simulink model "ADCS_Outline"  (R2019a)
settings: Solver=VariableStepAuto  StartTime=0.0  StopTime=duration  MaxStep=step
InitFcn:
  | SC_ODIN_INITIALIZATION
values from neighbouring files (symbols this model uses):
  A = [ v(1) v(4) v(5) v(7);        v(4) v(2) v(6) v(8);        v(5) v(6) v(3) v(9);        v(7) v(8) v(9) v(10) ]    [MagnetometerCalibration.m]    (also in SC_ODIN_INITIALIZATION.m = 0.06; test.m = asin(sin(N)/sin(n)*sin(a)))
  Amag = [0.910186583854  -0.00959593267728  0.00343590491018; -0.00959593267728  1.05471221352  0.0559849466324; 0.00343590491018  0.0559849466324  1.05528532305]    [MagnetometerBias.mat]    (also in MagnetometerCalibration.m = evecs/scale*evecs')
  argentina = [1612.36;-4182.16;-4522.83]    [SC_ODIN_INITIALIZATION.m]
  As = 0.2*0.3    (= 0.06)    [SC_ODIN_INITIALIZATION.m]
  b_mag = block.InputPort(3).Data    [MagnetometerCalibration.m]    (also in SC_ODIN_INITIALIZATION.m = [10;-15.5;-12.2]*1e-6)
  bmag = [1.00003671399e-05 -1.55007781395e-05 -1.22009762149e-05]    [MagnetometerBias.mat]    (also in MagnetometerCalibration.m = centerE)
  breakpoints = data(:,1)    [SC_ODIN_INITIALIZATION.m]
  c = 2.99792458e8    (= 299792458)    [SC_ODIN_INITIALIZATION.m]
  C_I = [0.045 0.0009 -0.00007;        0.0009 0.045 -0.00003;        -0.00007 -0.00003 0.009]    [SC_ODIN_INITIALIZATION.m]
  Cd = 2.0    (= 2)    [SC_ODIN_INITIALIZATION.m]
  controller_sample_rate = 0.5    [SC_ODIN_INITIALIZATION.m]
  D = [ 2 * x,            2 * y,            2 * z,            1 + 0 * x ]    [MagnetometerCalibration.m]    (also in SC_ODIN_INITIALIZATION.m = 0.01*[1;1;1])
  datapx = data(:,2)    [SC_ODIN_INITIALIZATION.m]
  datapy = data(:,3)    [SC_ODIN_INITIALIZATION.m]
  datapz = data(:,4)    [SC_ODIN_INITIALIZATION.m]
  datavx = data(:,5)    [SC_ODIN_INITIALIZATION.m]
  datavy = data(:,6)    [SC_ODIN_INITIALIZATION.m]
  datavz = data(:,7)    [SC_ODIN_INITIALIZATION.m]
  DCM_BT0 = eye(3)    [SC_ODIN_INITIALIZATION.m]
  G = 6.67408e-11    [SC_ODIN_INITIALIZATION.m]
  ground = [1266.06;-4295.81;4526.14]    [SC_ODIN_INITIALIZATION.m]
  I = [Ixx -Ixy -Ixz;      -Ixy Iyy -Iyz;      -Ixz -Iyz Izz]    [SC_ODIN_INITIALIZATION.m]
  invA_mag = block.InputPort(2).Data    [MagnetometerCalibration.m]    (also in SC_ODIN_INITIALIZATION.m = inv(Ellrot/scale*Ellrot'))
  JD_0 = start_day+start_fraction    [SC_ODIN_INITIALIZATION.m]
  Ks = 1367    [SC_ODIN_INITIALIZATION.m]
  L = [0.0000812 -0.0022136 -0.0225868]    [SC_ODIN_INITIALIZATION.m]
  Ls = 0.01*[-3; 3; 5]    [SC_ODIN_INITIALIZATION.m]
  M = 5.9722e24    (= 5.9722e+24)    [SC_ODIN_INITIALIZATION.m]    (also in visualisation.m = uicontrol('Style','text','String',{''},'Position',[710 100+2)
  magnetorquer_tau = 0.02    [SC_ODIN_INITIALIZATION.m]
  magnetorquer_x_saturation = 0.24    [SC_ODIN_INITIALIZATION.m]
  magnetorquer_y_saturation = 0.24    [SC_ODIN_INITIALIZATION.m]
  magnetorquer_z_saturation = 0.13    [SC_ODIN_INITIALIZATION.m]
  namibia = [5659.26;1238.85;-2659.2]    [SC_ODIN_INITIALIZATION.m]
  q = 0.6    [SC_ODIN_INITIALIZATION.m]
  radii = radii .* sgns    [MagnetometerCalibration.m]    (also in SC_ODIN_INITIALIZATION.m = [1;0.9;1.1])
  W0 = [1;0;1-1/240].*pi()/180    [SC_ODIN_INITIALIZATION.m]
  wheel_saturation = 0.23e-3    (= 0.00023)    [SC_ODIN_INITIALIZATION.m]
  wheel_tau = 2    [SC_ODIN_INITIALIZATION.m]
undefined symbols (not defined in the file or in its folder): DiscIntNeverNeededParam, nut80, sun_sensors
libraries: dspmathops x94, vrlib x70, dspsrcs4 x21, realtime_pacer_lib x1, dspsolvers x1, dspinverses x1
(part 1 of 6)
settings Model: ExtModeTrigDuration=2  Creator=Charles  LastModifiedBy=erinp
settings SolverCC: MaxConsecutiveMinStep=2  ZeroCrossControl=DisableAll  ZeroCrossAlgorithm=Adaptive
settings DataIOCC: ReturnWorkspaceOutputs=off
settings OptimizationCC: DefaultParameterBehavior=Inlined  EnhancedBackFolding=on  PassReuseOutputArgsAs=Individual arguments  MaxStackSize=64  OptimizeBlockOrder=speed  DifferentSizesBufferReuse=on  OptimizationCustomize=off
settings DebuggingCC: ReadBeforeWriteMsg=DisableAll  WriteAfterWriteMsg=DisableAll  WriteAfterReadMsg=DisableAll  IgnoredZcDiagnostic=none  MultiTaskDSMMsg=none  ParameterTunabilityLossMsg=error  ArithmeticOperatorsInVariantConditions=warning
settings HardwareCC: ProdBitPerInt=16  ProdBitPerPointer=16  ProdBitPerSizeT=16  ProdBitPerPtrDiffT=16  ProdLargestAtomicFloat=None  ProdWordSize=8  ProdHWDeviceType=Atmel->AVR  UseEmbeddedCoderFeatures=off  UseSimulinkCoderFeatures=off
settings ModelReferenceCC: UpdateModelReferenceTargets=IfOutOfDate
settings SFSimCC: SFSimEcho=off  MATLABDynamicMemAlloc=off
settings RTWCC: SystemTargetFile=ert.tlc  TemplateMakefile=ert_default_tmf  GenerateReport=on  Toolchain=Arduino AVR  BuildConfiguration=Faster Runs  IncludeHyperlinkInReport=on  LaunchReport=on  GenerateTraceInfo=on  GenerateTraceReport=on  GenerateTraceReportSl=on  GenerateTraceReportSf=on  GenerateTraceReportEml=on
settings CodeAppCC: ForceParamTrailComments=on  IgnoreCustomStorageClasses=off  OperatorAnnotations=on  SimulinkDataObjDesc=on  SFDataObjDesc=on  InsertBlockDesc=on
settings ERTTargetCC: SupportContinuousTime=on  SupportNonInlinedSFcns=on  ERTCustomFileTemplate=example_file_process.tlc

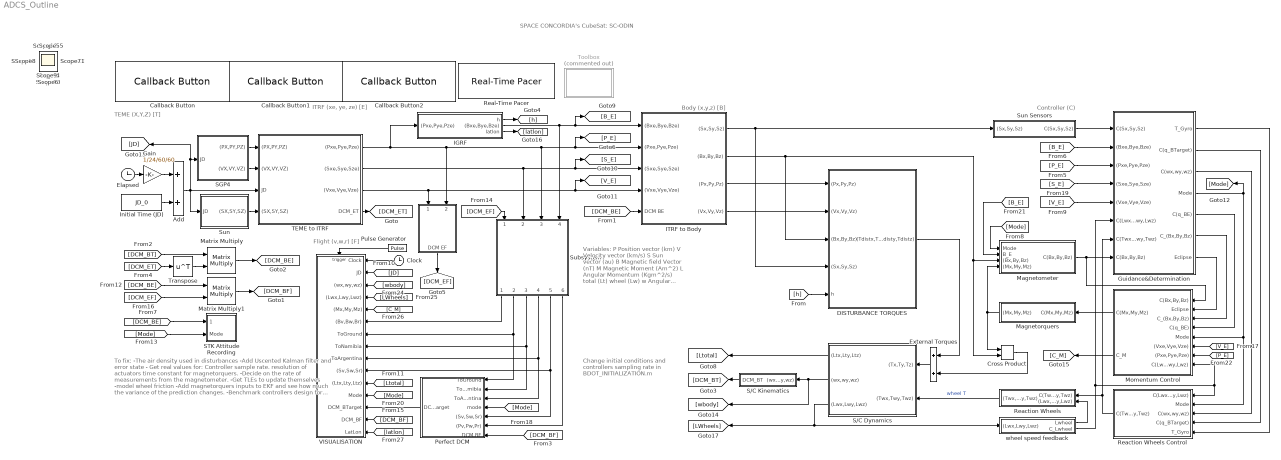
== system ADCS_Outline ==
  note: To fix:
      | -The air density used in disturbances
      | -Add Uscented Kalman filter and error state
      | - Get real values for:
      | Controller sample rate.
      | resolution of actuators
      | time constant for magnetorquers.
      | -Decide on the rate of measurements from the magnetometer.
      | -Get TLEs to update themselves
      | -model wheel friction
      | -Add magnetorquers inputs to EKF and see how much the variance of the prediction changes.
      | -Benchmark controllers design for other mission and see if ours makes sense.
      | -Get better estimate for center of mass from the Mech team
      | -Model vibrations from RWs with Vibs team
      | Stability: 0.01s picture. pixel = 3.2e-6 degrees
      |
      | -
      | -
  note: SPACE CONCORDIA's CubeSat: SC-ODIN
  note: Controller (C)
  note: Change initial conditions and controllers sampling rate in BDOT_INITIALIZATION.m
  note: Body (x,y,z) [B]
  note: Variables:
      |
      | P Position vector (km)
      | V Velocity vector (km/s)
      | S Sun vector (au)
      | B Magnetic field Vector (nT)
      | M Magnetic Moment (Am^2)
      | L Angular Momentum (Kgm^2/s)
      | total (Lt)
      | wheel (Lw)
      | w Angular velocity (rad/s)
      | T torque (Nm)
      | h Height from ground (km)
      | DCM Direction Cosine Matrix
  note: Flight (v,w,r) [F]
  note: TEME (X,Y,Z) [T]
  note: ITRF (xe, ye, ze) [E]
  "   " : Subsystem
  Add : Sum
  Callback Button : CallbackButton  ButtonText=Exclude visual
      settings: ClickFcn=|
      | if strcmp(get_param('ADCS_Outline/Callback Button','ButtonText'),'Include visual')
      | %un-comment visual related blocks
      | set_param('ADCS_Outline/Perfect DCM','Commented','off')
      | set_param('ADCS_Outline/VISUALISATION','Commented','off')
      | set_param('ADCS_Outline/From10','Commented','off')
      | set_param('ADCS_Outline/From11','Commented','off')
      | set_param('ADCS_Outline/From20','Commented','off')
      | set_param('ADCS_Outline/From15','Commented','off')
      | set_param('ADCS_Outline/From18','Commented','off')
      | set_param('ADCS_Outline/From3','Commented','off')
      | set_param('ADCS_Outline/   ','Commented','off')
      | set_param('ADCS_Outline/Goto5','Commented','off')
      | set_param('ADCS_Outline/Subsystem1','Commented','off')
      | set_param('ADCS_Outline/Subsystem1','Commented','off')
      | set_param('ADCS_Outline/Goto8','Commented','off')
      | set_param('ADCS_Outline/Matrix Multiply1','Commented','off')
      | set_param('ADCS_Outline/From12','Commented','off')
      | set_param('ADCS_Outline/From16','Commented','off')
      | set_param('ADCS_Outline/Goto1','Commented','off')
      | set_param('ADCS_Outline/From14','Commented','off')
      | set_param('ADCS_Outline/Goto13','Commented','off')
      | set_param('ADCS_Outline/From24','Commented','off')
      | set_param('ADCS_Outline/From25','Commented','off')
      | set_param('ADCS_Outline/From26','Commented','off')
      | set_param('ADCS_Outline/From27','Commented','off')
      | set_param('ADCS_Outline/Clock','Commented','off')
      | set_param('ADCS_Outline/Pulse Generator','Commented','off')
      | set_param('ADCS_Outline/Goto14','Commented','off')
      | set_param('ADCS_Outline/Goto15','Commented','off')
      | set_param('ADCS_Outline/Goto16','Commented','off')
      | set_param('ADCS_Outline/Goto17','Commented','off')
      | 
      | %change button text
      | set_param('ADCS_Outline/Callback Button','ButtonText','Exclude visual')
      | 
      | else
      | %comments out visual related blocks
      | set_param('ADCS_Outline/Perfect DCM','Commented','on')
      | set_param('ADCS_Outline/VISUALISATION','Commented','on')
      | set_param('ADCS_Outline/From10','Commented','on')
      | set_param('ADCS_Outline/From11','Commented','on')
      | set_param('ADCS_Outline/From20','Commented','on')
      | set_param('ADCS_Outline/From15','Commented','on')
      | set_param('ADCS_Outline/From18','Commented','on')
      | set_param('ADCS_Outline/From3','Commented','on')
      | set_param('ADCS_Outline/   ','Commented','on')
      | set_param('ADCS_Outline/Goto5','Commented','on')
      | set_param('ADCS_Outline/Subsystem1','Commented','on')
      | set_param('ADCS_Outline/Subsystem1','Commented','on')
      | set_param('ADCS_Outline/Goto8','Commented','on')
      | set_param('ADCS_Outline/Matrix Multiply1','Commented','on')
      | set_param('ADCS_Outline/From12','Commented','on')
      | set_param('ADCS_Outline/From16','Commented','on')
      | set_param('ADCS_Outline/Goto1','Commented','on')
      | set_param('ADCS_Outline/From14','Commented','on')
      | set_param('ADCS_Outline/Goto13','Commented','on')
      | set_param('ADCS_Outline/From24','Commented','on')
      | set_param('ADCS_Outline/From25','Commented','on')
      | set_param('ADCS_Outline/From26','Commented','on')
      | set_param('ADCS_Outline/From27','Commented','on')
      | set_param('ADCS_Outline/Clock','Commented','on')
      | set_param('ADCS_Outline/Pulse Generator','Commented','on')
      | set_param('ADCS_Outline/Goto14','Commented','on')
      | set_param('ADCS_Outline/Goto15','Commented','on')
      | set_param('ADCS_Outline/Goto16','Commented','on')
      | set_param('ADCS_Outline/Goto17','Commented','on')
      | 
      | %change button text
      | set_param('ADCS_Outline/Callback Button','ButtonText','Include visual')
      | end
  Callback Button1 : CallbackButton  ButtonText=Exclude STK Recording
      settings: ClickFcn=|
      | if strcmp(get_param('ADCS_Outline/Callback Button1','ButtonText'),'Include STK Recording')
      | %un-comment visual related blocks
      | set_param('ADCS_Outline/From7','Commented','off')
      | set_param('ADCS_Outline/From13','Commented','off')
      | set_param('ADCS_Outline/STK Attitude Recording','Commented','off')
      | 
      | %change button text
      | set_param('ADCS_Outline/Callback Button1','ButtonText','Exclude STK Recording')
      | 
      | else
      | %comments out visual related blocks
      | set_param('ADCS_Outline/From7','Commented','on')
      | set_param('ADCS_Outline/From13','Commented','on')
      | set_param('ADCS_Outline/STK Attitude Recording','Commented','on')
      | 
      | %change button text
      | set_param('ADCS_Outline/Callback Button1','ButtonText','Include STK Recording')
      | end
  Callback Button2 : CallbackButton  ButtonText=Exclude Momentum
      settings: ClickFcn=|
      | if strcmp(get_param('ADCS_Outline/Callback Button2','ButtonText'),'Include Momentum')
      | %un-comment visual related blocks
      | set_param('ADCS_Outline/Momentum Control','Commented','off')
      | set_param('ADCS_Outline/Magnetorquers','Commented','off')
      | set_param('ADCS_Outline/DISTURBANCE TORQUES','Commented','off')
      | set_param('ADCS_Outline/Cross Product','Commented','off')
      | set_param('ADCS_Outline/External Torques','Commented','off')
      | set_param('ADCS_Outline/From','Commented','off')
      | set_param('ADCS_Outline/Goto4','Commented','off')
      | 
      | %change button text
      | set_param('ADCS_Outline/Callback Button2','ButtonText','Exclude Momentum')
      | 
      | else
      | %comments out visual related blocks
      | set_param('ADCS_Outline/Momentum Control','Commented','on')
      | set_param('ADCS_Outline/Magnetorquers','Commented','on')
      | set_param('ADCS_Outline/DISTURBANCE TORQUES','Commented','on')
      | set_param('ADCS_Outline/Cross Product','Commented','on')
      | set_param('ADCS_Outline/External Torques','Commented','on')
      | set_param('ADCS_Outline/From','Commented','on')
      | set_param('ADCS_Outline/Goto4','Commented','on')
      | 
      | %change button text
      | set_param('ADCS_Outline/Callback Button2','ButtonText','Include Momentum')
      | end
  Clock : Clock
  Cross Product : vrlib/Utilities/Cross Product
      settings: SourceProductBaseCode=VR
  DISTURBANCE TORQUES : Subsystem
  Elapsed : Clock
  External Torques : Sum
  Gain : Gain  Gain=1/24/60/60
  Guidance&Determination : Subsystem  TreatAsAtomicUnit=on  SystemSampleTime=controller_sample_rate
  IGRF : Subsystem
  ITRF to Body : Subsystem
  Initial Time (JD) : Constant  Value=JD_0
  "Magnetometer " : Subsystem  TreatAsAtomicUnit=on  SystemSampleTime=controller_sample_rate
  Magnetorquers : Subsystem
  Matrix Multiply : Product  Multiplication=Matrix(*)
  Matrix Multiply1 : Product  Multiplication=Matrix(*)
  Momentum Control : Subsystem  TreatAsAtomicUnit=on  SystemSampleTime=controller_sample_rate/2
  Perfect DCM : Subsystem
  Pulse Generator : DiscretePulseGenerator  PulseType=Time based  Period=1  PulseWidth=5
  Reaction Wheels : Subsystem
  Reaction Wheels Control : Subsystem  TreatAsAtomicUnit=on  SystemSampleTime=controller_sample_rate
  Real-Time Pacer : realtime_pacer_lib/Real-Time Pacer  simTimePerRealTime=inf
  S/C Dynamics : Subsystem
  S/C Kinematics : Subsystem
  SGP4 : Subsystem
  STK Attitude Recording : Subsystem  StopFcn=STKAttitudeFileGenerator
  Subsystem1 : Subsystem
  Sun : Subsystem
  Sun Sensors : Subsystem  TreatAsAtomicUnit=on  SystemSampleTime=controller_sample_rate
  TEME to ITRF : Subsystem
  Toolbox : Subsystem  Commented=on
  Transpose : Math  Operator=transpose  SaturateOnIntegerOverflow=on
  VISUALISATION : Subsystem
  wheel speed feedback : Subsystem
  Scope{,1..10,12..21} (21 alike) : Scope
  wires:
  DISTURBANCE TORQUES/1((Tdistx,Tdisty,Tdistz)) -> External Torques/1
  ITRF to Body/3((Px,Py,Pz)) -> DISTURBANCE TORQUES/1((Px,Py,Pz))
  TEME to ITRF/3((Vxe,Vye,Vze)) -> ITRF to Body/4((Vxe,Vye,Vze)), [V_E], "   "/1((Vxe,Xye,Vze))
  Elapsed/1 -> Gain/1
  Gain/1 -> Add/1
  External Torques/1 -> S/C Dynamics/1((Tx,Ty,Tz))
  Initial Time (JD)/1 -> Add/2
  SGP4/2((VX,VY,VZ)) -> TEME to ITRF/2((VX,VY,VZ))
  SGP4/1((PX,PY,PZ)) -> TEME to ITRF/1((PX,PY,PZ))
  TEME to ITRF/2((Sxe,Sye,Sze)) -> ITRF to Body/3((Sxe,Sye,Sze)), [S_E], Subsystem1/2((Sxe,Sye,Sze))
  TEME to ITRF/4(DCM_ET) -> [DCM_ET]
  Matrix Multiply/1 -> [DCM_BE]
  IGRF/1("h ") -> [h]
  [h] -> DISTURBANCE TORQUES/5(h)
  [DCM_BT] -> Matrix Multiply/1
  [DCM_ET] -> Transpose/1
  Transpose/1 -> Matrix Multiply/2
  ITRF to Body/4((Vx,Vy,Vz)) -> DISTURBANCE TORQUES/2((Vx,Vy,Vz))
  TEME to ITRF/1((Pxe,Pye,Pze)) -> Subsystem1/3((Pxe,Pye,Pze)), ITRF to Body/2((Pxe,Pye,Pze)), [P_E], "   "/2((Pxe,Pye,Pze)), IGRF/1((Pxe,Pye,Pze))
  IGRF/2((Bxe,Bye,Bze)) -> Subsystem1/4((Bxe,Bye,Bze)), ITRF to Body/1((Bxe,Bye,Bze)), [B_E]
  Cross Product/1 -> External Torques/2
  Reaction Wheels Control/1(C(Twx,Twy,Twz)) -> Reaction Wheels/1(C(Twx,Twy,Twz)), Guidance&Determination/7(C(Twx,Twy,Twz))
  Reaction Wheels/1((Twx,Twy,Twz)) -> S/C Dynamics/2((Twx,Twy,Twz))  "wheel T"
  S/C Dynamics/3((Lwx,Lwy,Lwz)) -> wheel speed feedback/1((Lwx,Lwy,Lwz)), [LWheels]
  S/C Dynamics/1((Ltx,Lty,Ltz)) -> [Ltotal]
  "   "/1(DCM EF) -> [DCM_EF]
  [Ltotal] -> VISUALISATION/11((Ltx,Lty,Ltz))
  Momentum Control/1(C(Mx,My,Mz)) -> Magnetorquers/1(C(Mx,My,Mz))
  [DCM_EF] -> Matrix Multiply1/2
  [DCM_BE] -> Matrix Multiply1/1
  Matrix Multiply1/1 -> [DCM_BF]
  [DCM_EF] -> Subsystem1/1("DCM_EF ")
  [JD] -> VISUALISATION/2(JD)
  Subsystem1/1((Bv,Bw,Br)) -> VISUALISATION/6((Bv,Bw,Br))
  Sun Sensors/1(C(Sx,Sy,Sz)) -> Guidance&Determination/1(C(Sx,Sy,Sz))
  Subsystem1/2(ToGround) -> Perfect DCM/1(ToGround), VISUALISATION/7(ToGround)
  Subsystem1/5((Sv,Sw,Sr)) -> Perfect DCM/5((Sv,Sw,Sr)), VISUALISATION/10((Sv,Sw,Sr))
  [DCM_BF] -> VISUALISATION/14(DCM_BF)
  Sun/1((SX,SY,SZ)) -> TEME to ITRF/4((SX,SY,SZ))
  Perfect DCM/1(DCM BTarget) -> VISUALISATION/13(DCM_BTarget)
  [DCM_BF] -> Perfect DCM/7(DCM BF)
  Guidance&Determination/4(Mode) -> Reaction Wheels Control/2(Mode), Momentum Control/5(Mode), [Mode]
  [Mode] -> VISUALISATION/12(Mode)
  wheel speed feedback/2(C_Lwheel) -> Guidance&Determination/6(C(Lwx,Lwy,Lwz)), Momentum Control/8(C(Lwx,Lwy,Lwz)), Reaction Wheels Control/1(C(Lwx,Lwy,Lwz))
  Subsystem1/4(ToArgentina) -> Perfect DCM/3(ToArgentina), VISUALISATION/9(ToArgentina)
  Add/1 -> Sun/1(JD), SGP4/1(JD), [JD], TEME to ITRF/3(JD)
  [DCM_BE] -> STK Attitude Recording/1(DCM_BE)
  Subsystem1/3(ToNamibia) -> Perfect DCM/2(ToNamibia), VISUALISATION/8(ToNamibia)
  Subsystem1/6((Pv,Pw,Pr)) -> Perfect DCM/6((Pv,Pw,Pr))
  ITRF to Body/2((Bx,By,Bz)) -> DISTURBANCE TORQUES/3((Bx,By,Bz)), Cross Product/2, "Magnetometer "/3((Bx,By,Bz))
  Guidance&Determination/3(C(wx,wy,wz)) -> Reaction Wheels Control/3(C(wx,wy,wz))
  [Mode] -> STK Attitude Recording/2(Mode)
  ITRF to Body/1((Sx,Sy,Sz)) -> Sun Sensors/1((Sx,Sy,Sz)), DISTURBANCE TORQUES/4((Sx,Sy,Sz))
  [Mode] -> Perfect DCM/4(mode)
  [V_E] -> Momentum Control/6((Vxe,Vye,Vze))
  [P_E] -> Momentum Control/7((Pxe,Pye,Pze))
  [wbody] -> VISUALISATION/3((wx,wy,wz))
  [LWheels] -> VISUALISATION/4((Lwx,Lwy,Lwz))
  [C_M] -> VISUALISATION/5((Mx,My,Mz))
  Magnetorquers/1((Mx,My,Mz)) -> "Magnetometer "/4((Mx,My,Mz)), Cross Product/1
  Momentum Control/2(C_M) -> [C_M]
  IGRF/3(latlon) -> [latlon]
  [latlon] -> VISUALISATION/15(LatLon)
  Pulse Generator/1 -> VISUALISATION/Trigger
  Clock/1 -> VISUALISATION/1(Clock)
  Guidance&Determination/2(C(q_BTarget)) -> Reaction Wheels Control/4(C(q_BTarget))
  Guidance&Determination/5(C(q_BE)) -> Momentum Control/4(C(q_BE))
  Guidance&Determination/6(C_(Bx,By,Bz)) -> Momentum Control/3(C_(Bx,By,Bz))
  "Magnetometer "/1(C(Bx,By,Bz)) -> Guidance&Determination/8(C(Bx,By,Bz)), Momentum Control/1(C(Bx,By,Bz))
  wheel speed feedback/1(Lwheel) -> Reaction Wheels/2((Lwx,Lwy,Lwz))
  [Mode] -> "Magnetometer "/1(Mode)
  S/C Kinematics/1(DCM_BT) -> [DCM_BT]
  Guidance&Determination/7(Eclipse) -> Momentum Control/2(Eclipse)
  S/C Dynamics/2((wx,wy,wz)) -> S/C Kinematics/1(" (wx,wy,wz)"), [wbody]
  [DCM_BE] -> ITRF to Body/5(DCM BE)
  [B_E] -> "Magnetometer "/2(B_E)
  [B_E] -> Guidance&Determination/2((Bxe,Bye,Bze))
  [P_E] -> Guidance&Determination/3((Pxe,Pye,Pze))
  [S_E] -> Guidance&Determination/4((Sxe,Sye,Sze))
  [V_E] -> Guidance&Determination/5((Vxe,Vye,Vze))
  Guidance&Determination/1(T_Gyro) -> Reaction Wheels Control/5(T_Gyro)

== system ADCS_Outline/    ==
  (Vxe,Xye,Vze) : Inport
  (Pxe,Pye,Pze) : Inport  Port=2
  Constant : Constant  Value=[1;0;0]
  Constant1 : Constant  Value=[0;0;1]
  Cross Product{,1..3} (4 alike) : vrlib/Utilities/Cross Product
      settings: SourceProductBaseCode=VR
  Matrix Concatenate : Concatenate  NumInputs=3  Mode=Multidimensional array  ConcatenateDimension=2
  Matrix Concatenate1 : Concatenate  NumInputs=3  Mode=Multidimensional array  ConcatenateDimension=2
  Matrix Multiply : Product  Multiplication=Matrix(*)
  Normalization{,1..5} (6 alike) : dspmathops/Normalization  NormType=2-norm  Bias=1e-10  NormOver=Each column  Dimension=1  roundingMode=Floor  overflowMode=off  accumDataTypeStr=Inherit: Same as product output  accumLastDataTypeStr=Inherit: Same as product output  outputDataTypeStr=Inherit: Same as product output  outputMin=[]  outputMax=[]  outputLastDataTypeStr=Inherit: Same as product output
      settings: SourceProductName=DSP System Toolbox
  Signal Specification1 : SignalSpecification  Dimensions=3
  Transpose : Math  Operator=transpose  SaturateOnIntegerOverflow=on
  DCM EF : Outport
  wires:
  Normalization/1 -> Matrix Concatenate/3, Cross Product1/1
  Normalization5/1 -> Matrix Concatenate1/1, Cross Product3/2
  Cross Product1/1 -> Normalization1/1
  Normalization3/1 -> Matrix Concatenate1/2
  Cross Product3/1 -> Signal Specification1/1
  Constant1/1 -> Cross Product/2
  Normalization4/1 -> Matrix Concatenate/1, Cross Product1/2
  Constant/1 -> Normalization4/1, Cross Product/1
  Cross Product2/1 -> Normalization2/1
  Cross Product/1 -> Normalization/1
  Normalization1/1 -> Matrix Concatenate/2
  Normalization2/1 -> Cross Product3/1, Matrix Concatenate1/3
  Matrix Concatenate/1 -> Transpose/1
  Matrix Concatenate1/1 -> Matrix Multiply/1
  Transpose/1 -> Matrix Multiply/2
  (Vxe,Xye,Vze)/1 -> Cross Product2/1, Normalization5/1
  (Pxe,Pye,Pze)/1 -> Cross Product2/2
  Matrix Multiply/1 -> DCM EF/1
  Signal Specification1/1 -> Normalization3/1

== system ADCS_Outline/DISTURBANCE TORQUES ==
  note: DISTURBANCE TORQUE
  (Px,Py,Pz) : Inport
  (Vx,Vy,Vz) : Inport  Port=2
  (Bx,By,Bz) : Inport  Port=3
  (Sx,Sy,Sz) : Inport  Port=4
  h : Inport  Port=5
  ATMOSPHERIC DRAG : Subsystem
  GRAVITY GRADIENT : Subsystem
  Inertia Matrix : Constant  Value=I
  "MAGNETIC FIELD " : Subsystem
  S/C residual Dipole Moment : Constant  Value=D
  SOLAR RADIATION PRESSURE : Subsystem
  Scope : Scope  NumInputPorts=4
  Sum : Sum  Inputs=++++
  (Tdistx,Tdisty,Tdistz) : Outport
  wires:
  (Px,Py,Pz)/1 -> GRAVITY GRADIENT/1((px,py,pz))
  (Sx,Sy,Sz)/1 -> SOLAR RADIATION PRESSURE/1((Sx,Sy,Sz))
  Inertia Matrix/1 -> GRAVITY GRADIENT/2("(Ixx Ixy Ixz, Iyx Iyy Iyz, Izx Izy Izz)")
  (Vx,Vy,Vz)/1 -> ATMOSPHERIC DRAG/1((vx,vy,vz))
  (Bx,By,Bz)/1 -> "MAGNETIC FIELD "/2((Bx,By,Bz))
  S/C residual Dipole Moment/1 -> "MAGNETIC FIELD "/1((Dx,Dy,Dz))
  "MAGNETIC FIELD "/1((Tmx,Tmy,Tmz)) -> Scope/1, Sum/1
  GRAVITY GRADIENT/1((Tgx,Tgy,Tgz)) -> Scope/2, Sum/2
  SOLAR RADIATION PRESSURE/1("(Tsx,Tsy, Tsz)") -> Scope/3, Sum/3
  ATMOSPHERIC DRAG/1((Tax,Tay,Taz)) -> Scope/4, Sum/4
  h/1 -> ATMOSPHERIC DRAG/2("h ")
  Sum/1 -> (Tdistx,Tdisty,Tdistz)/1

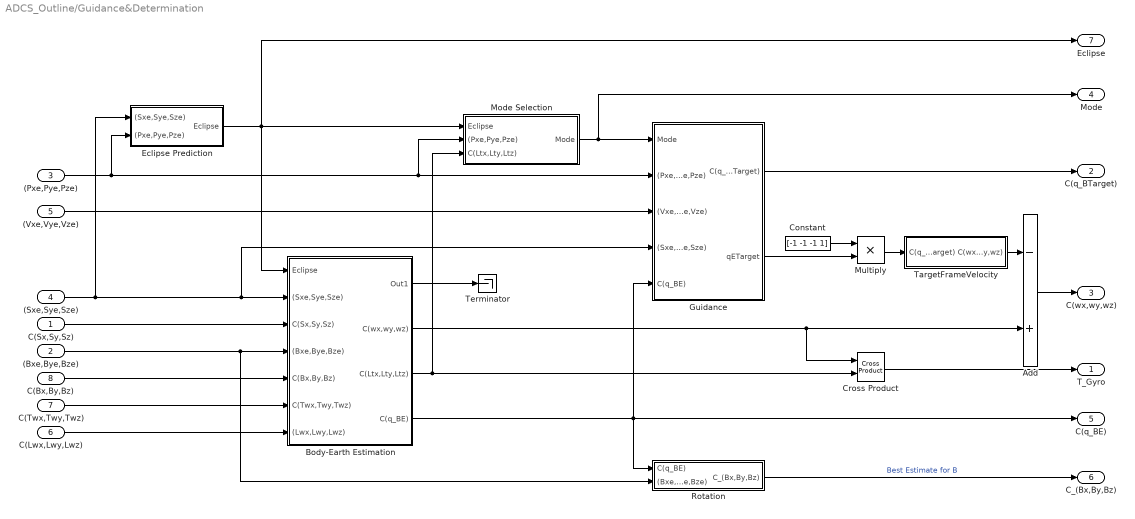
== system ADCS_Outline/Guidance&Determination ==
  C(Sx,Sy,Sz) : Inport
  (Bxe,Bye,Bze) : Inport  Port=2
  (Pxe,Pye,Pze) : Inport  Port=3
  (Sxe,Sye,Sze) : Inport  Port=4
  (Vxe,Vye,Vze) : Inport  Port=5
  C(Lwx,Lwy,Lwz) : Inport  Port=6
  C(Twx,Twy,Twz) : Inport  Port=7
  C(Bx,By,Bz) : Inport  Port=8
  Add : Sum  Inputs=-+
  Body-Earth Estimation : Subsystem
  Constant : Constant  Value=[-1 -1 -1 1]
  Cross Product : vrlib/Utilities/Cross Product
      settings: SourceProductBaseCode=VR
  Eclipse Prediction : Subsystem
  Guidance : Subsystem
  Mode Selection : Subsystem
  Multiply : Product
  Rotation : Subsystem
  TargetFrameVelocity : Subsystem
  Terminator : Terminator
  T_Gyro : Outport
  C(q_BTarget) : Outport  Port=2
  C(wx,wy,wz) : Outport  Port=3
  Mode : Outport  Port=4
  C(q_BE) : Outport  Port=5
  C_(Bx,By,Bz) : Outport  Port=6
  Eclipse : Outport  Port=7
  wires:
  (Bxe,Bye,Bze)/1 -> Body-Earth Estimation/4((Bxe,Bye,Bze)), Rotation/2((Bxe,Bye,Bze))
  (Sxe,Sye,Sze)/1 -> Eclipse Prediction/1((Sxe,Sye,Sze)), Guidance/4((Sxe,Sye,Sze)), Body-Earth Estimation/2((Sxe,Sye,Sze))
  (Pxe,Pye,Pze)/1 -> Eclipse Prediction/2((Pxe,Pye,Pze)), Mode Selection/2((Pxe,Pye,Pze)), Guidance/2((Pxe,Pye,Pze))
  C(Lwx,Lwy,Lwz)/1 -> Body-Earth Estimation/7((Lwx,Lwy,Lwz))
  C(Sx,Sy,Sz)/1 -> Body-Earth Estimation/3(C(Sx,Sy,Sz))
  C(Twx,Twy,Twz)/1 -> Body-Earth Estimation/6(C(Twx,Twy,Twz))
  Body-Earth Estimation/4(C(q_BE)) -> Guidance/5(C(q_BE)), C(q_BE)/1, Rotation/1(C(q_BE))
  (Vxe,Vye,Vze)/1 -> Guidance/3((Vxe,Vye,Vze))
  Guidance/1(C(q_BTarget)) -> C(q_BTarget)/1
  Mode Selection/1(Mode) -> Mode/1, Guidance/1(Mode)
  Body-Earth Estimation/3(C(Ltx,Lty,Ltz)) -> Mode Selection/3(C(Ltx,Lty,Ltz)), Cross Product/2
  Rotation/1(C_(Bx,By,Bz)) -> C_(Bx,By,Bz)/1  "Best Estimate for B"
  C(Bx,By,Bz)/1 -> Body-Earth Estimation/5(C(Bx,By,Bz))
  Eclipse Prediction/1(Eclipse) -> Body-Earth Estimation/1(Eclipse), Eclipse/1, Mode Selection/1(Eclipse)
  Add/1 -> C(wx,wy,wz)/1
  Body-Earth Estimation/2(C(wx,wy,wz)) -> Cross Product/1, Add/2
  Constant/1 -> Multiply/1
  Guidance/2(qETarget) -> Multiply/2
  TargetFrameVelocity/1(C(wx,wy,wz)) -> Add/1
  Multiply/1 -> TargetFrameVelocity/1(C(q_ETarget))
  Body-Earth Estimation/1(Out1) -> Terminator/1
  Cross Product/1 -> T_Gyro/1

== system ADCS_Outline/IGRF ==
  note: NED (n,e,d)
  (Pxe,Pye,Pze) : Inport
  Demux : Demux  Outputs=3
  Dot Product : DotProduct  InputSameDT=on  OutDataTypeStr=Inherit: Inherit via internal rule
  Gain : Gain  Gain=-1
  Gain1 : Gain  Gain=1e-9
  MATLAB Function : MATLAB Function  TreatAsAtomicUnit=on
  MATLAB Function1 : MATLAB Function  TreatAsAtomicUnit=on
  MATLAB Function2 : MATLAB Function  TreatAsAtomicUnit=on
  Mux : Mux  Inputs=3
  Mux1 : Mux  Inputs=2
  Scope : Scope
  Sqrt : Sqrt  SaturateOnIntegerOverflow=on
  km to m : Gain  Gain=1000
  m to km : Gain  Gain=1/1000
  m2km : Gain  Gain=1/1000
  "h " : Outport
  (Bxe,Bye,Bze) : Outport  Port=2
  latlon : Outport  Port=3
  wires:
  MATLAB Function/1(Bn) -> MATLAB Function2/1(dx)
  MATLAB Function/2(Be) -> MATLAB Function2/2(dy)
  MATLAB Function1/2(lon) -> Mux1/2, MATLAB Function2/5(lon), MATLAB Function/2(longitude)
  MATLAB Function1/1(lat) -> Mux1/1, MATLAB Function2/4(lat), MATLAB Function/1(latitude)
  MATLAB Function1/3(altitude) -> m to km/1  "m"
  (Pxe,Pye,Pze)/1 -> km to m/1
  km to m/1 -> Demux/1
  Demux/3 -> MATLAB Function1/3(Z)
  Demux/2 -> MATLAB Function1/2(Y)
  Demux/1 -> MATLAB Function1/1(X)
  m to km/1 -> MATLAB Function/3(altitude)
  MATLAB Function2/3(dZ) -> Mux/3
  MATLAB Function2/1(dX) -> Mux/1
  MATLAB Function2/2(dY) -> Mux/2
  MATLAB Function/3(Bd) -> Gain/1
  Gain/1 -> MATLAB Function2/3(dz)
  MATLAB Function1/4(h) -> m2km/1
  m2km/1 -> "h "/1
  Mux/1 -> Gain1/1
  Mux1/1 -> latlon/1
  Gain1/1 -> Dot Product/1, Dot Product/2, (Bxe,Bye,Bze)/1
  Dot Product/1 -> Sqrt/1
  Sqrt/1 -> Scope/1

== system ADCS_Outline/ITRF to Body ==
  (Bxe,Bye,Bze) : Inport
  (Pxe,Pye,Pze) : Inport  Port=2
  (Sxe,Sye,Sze) : Inport  Port=3
  (Vxe,Vye,Vze) : Inport  Port=4
  DCM BE : Inport  Port=5
  Angle between vectors : MATLAB Function  TreatAsAtomicUnit=on
  Constant : Constant  Value=[0;0;0]
  Matrix Multiply{2..5} (4 alike) : Product  Multiplication=Matrix(*)
  Switch : Switch  Criteria=u2 > Threshold  Threshold=109.79
  (Sx,Sy,Sz) : Outport
  (Bx,By,Bz) : Outport  Port=2
  (Px,Py,Pz) : Outport  Port=3
  (Vx,Vy,Vz) : Outport  Port=4
  wires:
  (Bxe,Bye,Bze)/1 -> Matrix Multiply5/2
  DCM BE/1 -> Matrix Multiply4/1, Matrix Multiply3/1, Matrix Multiply2/1, Matrix Multiply5/1
  Matrix Multiply5/1 -> (Bx,By,Bz)/1
  (Pxe,Pye,Pze)/1 -> Angle between vectors/2(v), Matrix Multiply3/2
  Matrix Multiply3/1 -> (Px,Py,Pz)/1
  Matrix Multiply4/1 -> Switch/3
  (Sxe,Sye,Sze)/1 -> Angle between vectors/1(u), Matrix Multiply4/2
  (Vxe,Vye,Vze)/1 -> Matrix Multiply2/2
  Matrix Multiply2/1 -> (Vx,Vy,Vz)/1
  Switch/1 -> (Sx,Sy,Sz)/1
  Angle between vectors/1(y) -> Switch/2
  Constant/1 -> Switch/1

== system ADCS_Outline/Magnetometer  ==
  note: Residual moment interference with magnetometer needs to be researched
  Mode : Inport
  B_E : Inport  Port=2
  (Bx,By,Bz) : Inport  Port=3
  (Mx,My,Mz) : Inport  Port=4
  Add : Sum
  Calibration (Calculated onboard) : Subsystem
  Delay One Step : Delay  DelayLength=1
  Gain : Gain  Commented=on  Gain=1e-2
  Noise and Bias : Subsystem
  C(Bx,By,Bz) : Outport
  wires:
  (Mx,My,Mz)/1 -> Gain/1
  (Bx,By,Bz)/1 -> Add/1
  Gain/1 -> Add/2
  Mode/1 -> Delay One Step/1
  Delay One Step/1 -> Calibration (Calculated onboard)/2(Mode)
  Add/1 -> Noise and Bias/1(In1)
  Noise and Bias/1(Out1) -> Calibration (Calculated onboard)/1(C(Bx,By,Bz)raw)
  Calibration (Calculated onboard)/1(C(Bx,By,Bz)cal) -> C(Bx,By,Bz)/1
  B_E/1 -> Calibration (Calculated onboard)/3(B_E)

== system ADCS_Outline/Magnetorquers ==
  note: more accurate
  note: makes the simulation SO much faster, the precision of the magnetometer response is not critical for most simulation usage
  C(Mx,My,Mz) : Inport
  Add : Sum  Commented=on
  Demux : Demux  Commented=on  Outputs=3
  Mux : Mux  Commented=on  Inputs=3
  Residual Dipole : Constant  Commented=on  Value=[1;1;1]*1e-2
  Saturation : Saturate  Commented=on  UpperLimit=magnetorquer_x_saturation  LowerLimit=-magnetorquer_x_saturation  ZeroCross=off
  Saturation1 : Saturate  Commented=on  UpperLimit=magnetorquer_y_saturation  LowerLimit=-magnetorquer_y_saturation  ZeroCross=off
  Saturation2 : Saturate  Commented=on  UpperLimit=magnetorquer_z_saturation  LowerLimit=-magnetorquer_z_saturation  ZeroCross=off
  Transfer Fcn1 : TransferFcn  Commented=on  Numerator=[1/magnetorquer_tau]  Denominator=[1 1/magnetorquer_tau]
  Transfer Fcn2 : TransferFcn  Commented=on  Numerator=[1/magnetorquer_tau]  Denominator=[1 1/magnetorquer_tau]
  Transfer Fcn3 : TransferFcn  Commented=on  Numerator=[1/magnetorquer_tau]  Denominator=[1 1/magnetorquer_tau]
  (Mx,My,Mz) : Outport
  wires:
  Demux/3 -> Transfer Fcn2/1
  Demux/2 -> Transfer Fcn1/1
  Demux/1 -> Transfer Fcn3/1
  Transfer Fcn1/1 -> Saturation1/1
  Transfer Fcn3/1 -> Saturation/1
  Transfer Fcn2/1 -> Saturation2/1
  Saturation/1 -> Mux/1
  Saturation1/1 -> Mux/2
  Saturation2/1 -> Mux/3
  Mux/1 -> Add/2
  Residual Dipole/1 -> Add/1
  C(Mx,My,Mz)/1 -> (Mx,My,Mz)/1, Demux/1

== system ADCS_Outline/Momentum Control ==
  C(Bx,By,Bz) : Inport
  Eclipse : Inport  Port=2
  C_(Bx,By,Bz) : Inport  Port=3
  C(q_BE) : Inport  Port=4
  Mode : Inport  Port=5
  (Vxe,Vye,Vze) : Inport  Port=6
  (Pxe,Pye,Pze) : Inport  Port=7
  C(Lwx,Lwy,Lwz) : Inport  Port=8
  Add : Sum  Inputs=-+
  Bdot Controller : Subsystem
  Control Gain : Gain  Gain=-1e6
  Cross Product : vrlib/Utilities/Cross Product
      settings: SourceProductBaseCode=VR
  Filter : Subsystem
  Momentum Bias : Subsystem
  Saturation : Subsystem
  Switch : MATLAB Function  TreatAsAtomicUnit=on
  C(Mx,My,Mz) : Outport
  C_M : Outport  Port=2
  wires:
  C_(Bx,By,Bz)/1 -> Cross Product/1
  Control Gain/1 -> Saturation/1(C(Mx,My,Mz))
  Mode/1 -> Switch/1(Mode)
  Bdot Controller/1(C(Mx,My,Mz)) -> Switch/3(Bdot)
  Saturation/1(sat_C(Mx,My,Mz)) -> Switch/4(Nominal)
  C(Lwx,Lwy,Lwz)/1 -> Add/2
  Switch/2(M) -> C(Mx,My,Mz)/1
  Switch/1(CM) -> C_M/1
  C(q_BE)/1 -> Momentum Bias/1(C(q_BE))
  (Vxe,Vye,Vze)/1 -> Momentum Bias/2((Vxe,Vye,Vze))
  (Pxe,Pye,Pze)/1 -> Momentum Bias/3((Pxe,Pye,Pze))
  Add/1 -> Cross Product/2
  Cross Product/1 -> Filter/1(Noisy)
  Momentum Bias/1(C(M_B)) -> Add/1
  Filter/1(Filtered) -> Control Gain/1
  C(Bx,By,Bz)/1 -> Bdot Controller/1(C(Bx,By,Bz))
  Eclipse/1 -> Switch/2(Eclipse)

== system ADCS_Outline/Perfect DCM ==
  ToGround : Inport
  ToNamibia : Inport  Port=2
  ToArgentina : Inport  Port=3
  mode : Inport  Port=4
  (Sv,Sw,Sr) : Inport  Port=5
  (Pv,Pw,Pr) : Inport  Port=6
  DCM BF : Inport  Port=7
  " Imaging Argentina" : Subsystem
  " Imaging Namibia" : Subsystem
  " Nadir Pointing" : Subsystem
  Gound Station Pointing : Subsystem
  Mode Selection : MATLAB Function  TreatAsAtomicUnit=on
  Sun Pointing : Subsystem
  DCM BTarget : Outport
  wires:
  (Sv,Sw,Sr)/1 -> Sun Pointing/1((Sv,Sw,Sr))
  Sun Pointing/1(DCM FS) -> Mode Selection/3(DCM_S)
  Gound Station Pointing/1(DCM FG) -> Mode Selection/4(DCM_G)
  ToGround/1 -> Gound Station Pointing/1(ToGround)
  ToArgentina/1 -> " Imaging Argentina"/1(ToArgentina)
  " Imaging Argentina"/1(DCM FN) -> Mode Selection/5(DCM_A)
  " Imaging Namibia"/1(DCM FN) -> Mode Selection/6(DCM_N)
  ToNamibia/1 -> " Imaging Namibia"/1(ToNamibia)
  (Pv,Pw,Pr)/1 -> " Nadir Pointing"/1((Pv,Pw,Pr))
  " Nadir Pointing"/1(DCM FZ) -> Mode Selection/7(DCM_Z)
  Mode Selection/1(DCM_BTarget) -> DCM BTarget/1
  DCM BF/1 -> Mode Selection/1(DCM_BF)
  mode/1 -> Mode Selection/2(Mode)

== system ADCS_Outline/Reaction Wheels ==
  C(Twx,Twy,Twz) : Inport
  (Lwx,Lwy,Lwz) : Inport  Port=2
  Add : Sum
  Friction : Gain  Commented=on  Gain=-0.01
  MATLAB Function : MATLAB Function  TreatAsAtomicUnit=on
  Torque Saturation : Subsystem
  (Twx,Twy,Twz) : Outport
  wires:
  (Lwx,Lwy,Lwz)/1 -> Friction/1, MATLAB Function/2(Lw)
  Add/1 -> (Twx,Twy,Twz)/1
  MATLAB Function/1(Tw) -> Torque Saturation/1(C(Twx,Twy,Twz))
  Friction/1 -> Add/2
  C(Twx,Twy,Twz)/1 -> MATLAB Function/1(Ti)
  Torque Saturation/1(sat_C(Twx,Twy,Twz)) -> Add/1

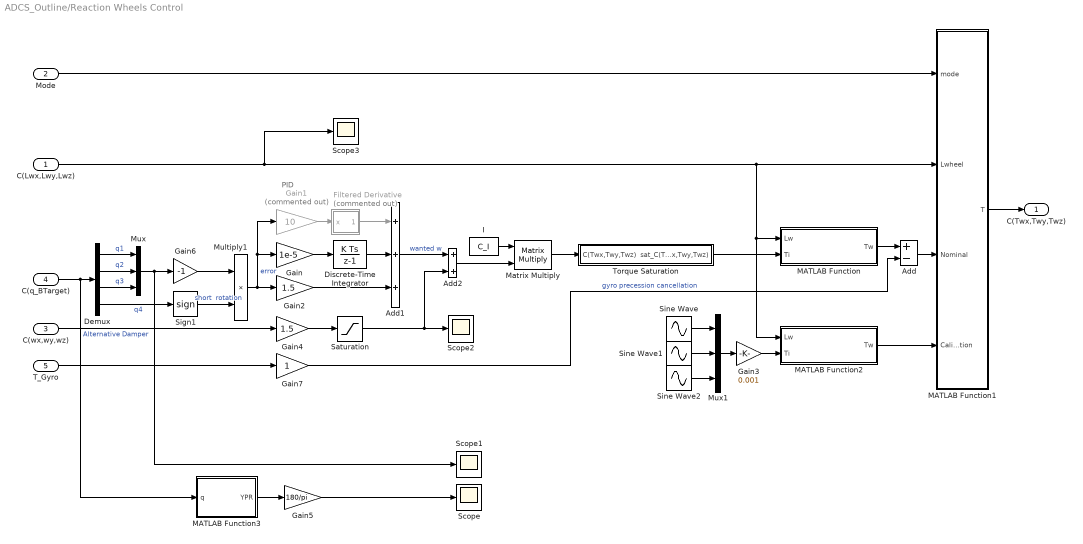
== system ADCS_Outline/Reaction Wheels Control ==
  note: PID
  C(Lwx,Lwy,Lwz) : Inport
  Mode : Inport  Port=2
  C(wx,wy,wz) : Inport  Port=3
  C(q_BTarget) : Inport  Port=4
  T_Gyro : Inport  Port=5
  Add : Sum  Inputs=+-
  Add1 : Sum  Inputs=3
  Add2 : Sum
  Demux : Demux
  Discrete-Time Integrator : DiscreteIntegrator  SampleTime=-1  ICPrevOutput=DiscIntNeverNeededParam  ICPrevScaledInput=DiscIntNeverNeededParam
  Filtered Derivative : Subsystem  Commented=on
  Gain : Gain  Gain=1e-5
  Gain1 : Gain  Commented=on  Gain=10
  Gain2 : Gain  Gain=1.5
  Gain3 : Gain  Gain=0.001
  Gain4 : Gain  Gain=1.5
  Gain5 : Gain  Gain=180/pi
  Gain6 : Gain  Gain=-1
  Gain7 : Gain
  I : Constant  Value=C_I
  MATLAB Function : MATLAB Function  TreatAsAtomicUnit=on
  MATLAB Function1 : MATLAB Function  TreatAsAtomicUnit=on
  MATLAB Function2 : MATLAB Function  TreatAsAtomicUnit=on
  MATLAB Function3 : MATLAB Function  TreatAsAtomicUnit=on
  Matrix Multiply : Product  Multiplication=Matrix(*)
  Multiply1 : Product
  Mux : Mux  Inputs=3
  Mux1 : Mux  Inputs=3
  Saturation : Saturate  UpperLimit=0.08  LowerLimit=-0.08
  Scope{,1..3} (4 alike) : Scope
  Sign1 : Signum
  Sine Wave : Sin  Amplitude=0.1  Frequency=0.006  Phase=1
  Sine Wave1 : Sin  Amplitude=0.1  Frequency=0.011  Phase=2
  Sine Wave2 : Sin  Amplitude=0.05  Frequency=0.05  Phase=3
  Torque Saturation : Subsystem
  C(Twx,Twy,Twz) : Outport
  wires:
  Multiply1/1 -> Gain/1, Gain1/1, Gain2/1  "error"
  Filtered Derivative/1(dx) -> Add1/1
  Gain1/1 -> Filtered Derivative/1(x)
  Demux/1 -> Mux/1  "q1"
  Mux/1 -> Scope1/1, Gain6/1
  Add1/1 -> Add2/1  "wanted w"
  Gain4/1 -> Saturation/1
  Sign1/1 -> Multiply1/2  "short  rotation"
  C(Lwx,Lwy,Lwz)/1 -> Scope3/1, MATLAB Function1/2(Lwheel), MATLAB Function/1(Lw), MATLAB Function2/1(Lw)
  C(wx,wy,wz)/1 -> Gain4/1  "Alternative Damper"
  Mode/1 -> MATLAB Function1/1(mode)
  MATLAB Function1/1(T) -> C(Twx,Twy,Twz)/1
  C(q_BTarget)/1 -> MATLAB Function3/1(q), Demux/1
  I/1 -> Matrix Multiply/1
  Demux/2 -> Mux/2  "q2"
  Demux/3 -> Mux/3  "q3"
  Demux/4 -> Sign1/1  "q4"
  Sine Wave/1 -> Mux1/1
  Sine Wave2/1 -> Mux1/3
  Sine Wave1/1 -> Mux1/2
  MATLAB Function2/1(Tw) -> MATLAB Function1/4(Calibration)
  Mux1/1 -> Gain3/1
  Gain3/1 -> MATLAB Function2/2(Ti)
  MATLAB Function3/1(YPR) -> Gain5/1
  Gain5/1 -> Scope/1
  Gain6/1 -> Multiply1/1
  Discrete-Time Integrator/1 -> Add1/2
  Gain/1 -> Discrete-Time Integrator/1
  T_Gyro/1 -> Gain7/1
  Matrix Multiply/1 -> Torque Saturation/1(C(Twx,Twy,Twz))
  Add2/1 -> Matrix Multiply/2
  Torque Saturation/1(sat_C(Twx,Twy,Twz)) -> MATLAB Function/2(Ti)
  Saturation/1 -> Scope2/1, Add2/2
  MATLAB Function/1(Tw) -> Add/1
  Add/1 -> MATLAB Function1/3(Nominal)
  Gain7/1 -> Add/2  "gyro precession cancellation"
  Gain2/1 -> Add1/3

== system ADCS_Outline/S//C Dynamics ==
  (Tx,Ty,Tz) : Inport
  (Twx,Twy,Twz) : Inport  Port=2
  Add : Sum  Inputs=-+-
  Add1 : Sum
  Add2 : Sum  Inputs=+-
  Constant : Constant  Value=[0;0;0]
  Cross Product : vrlib/Utilities/Cross Product
      settings: SourceProductBaseCode=VR
  Gain : Gain  Gain=1/100
  Inertia matrix I : Constant  Value=I
  Initial Angular Velocity : Constant  Value=W0
  Integrator : Integrator  InitialConditionSource=external
  Integrator1 : Integrator  InitialConditionSource=external
  Inverse of I : Constant  Value=inv(I)
  "Inverse of I " : Constant  Value=inv(I)
  J_wheel : Gain  Gain=2.11e-6
  Matrix Multiply : Product  Multiplication=Matrix(*)
  Matrix Multiply1 : Product  Multiplication=Matrix(*)
  Matrix Multiply2 : Product  Multiplication=Matrix(*)
  Scope : Scope  NumInputPorts=2
  (Ltx,Lty,Ltz) : Outport
  (wx,wy,wz) : Outport  Port=2
  (Lwx,Lwy,Lwz) : Outport  Port=3
  wires:
  Add/1 -> Scope/1, Matrix Multiply2/2, Integrator/1  "I*w_dot"
  Cross Product/1 -> Add/3
  Integrator/1 -> Add1/2, Matrix Multiply/2  "I*w SC L"
  Inverse of I/1 -> Matrix Multiply/1
  Inertia matrix I/1 -> Matrix Multiply1/1
  Matrix Multiply/1 -> Gain/1, (wx,wy,wz)/1, Cross Product/1  "w"
  Matrix Multiply1/1 -> Integrator/2
  (Tx,Ty,Tz)/1 -> Add/2
  Initial Angular Velocity/1 -> Matrix Multiply1/2
  (Twx,Twy,Twz)/1 -> Add/1, Add2/1
  J_wheel/1 -> Add2/2
  Add2/1 -> Integrator1/1
  Integrator1/1 -> Add1/1, (Lwx,Lwy,Lwz)/1  "I*wh Wheels Lw"
  Matrix Multiply2/1 -> J_wheel/1
  "Inverse of I "/1 -> Matrix Multiply2/1
  Add1/1 -> (Ltx,Lty,Ltz)/1, Cross Product/2
  Constant/1 -> Integrator1/2
  Gain/1 -> Scope/2

== system ADCS_Outline/S//C Kinematics ==
  note: Cdot=-wxC
  " (wx,wy,wz)" : Inport
  Gain : Gain  Gain=-1
  Initial attitude : Constant  Value=DCM_BT0
  Integrator : Integrator  InitialConditionSource=external
  Matrix Multiply : Product  Multiplication=Matrix(*)
  Skewed : Subsystem
  DCM_BT : Outport
  wires:
  Matrix Multiply/1 -> Integrator/1
  Skewed/1(m) -> Matrix Multiply/1
  Initial attitude/1 -> Integrator/2
  Integrator/1 -> DCM_BT/1, Matrix Multiply/2
  " (wx,wy,wz)"/1 -> Gain/1
  Gain/1 -> Skewed/1(v)

== system ADCS_Outline/SGP4 ==
  JD : Inport
  Mux : Mux  Inputs=3
  Mux1 : Mux  Inputs=3
  PX : Lookup_n-D  NumberOfTableDimensions=1  BreakpointsForDimension1=breakpoints  BeginIndexSearchUsingPreviousIndexResult=on  Table=datapx  InterpMethod=Cubic spline  InternalRulePriority=Speed  RndMeth=Simplest  InputSameDT=on
  PY : Lookup_n-D  NumberOfTableDimensions=1  BreakpointsForDimension1=breakpoints  BeginIndexSearchUsingPreviousIndexResult=on  Table=datapy  InterpMethod=Cubic spline  InternalRulePriority=Speed  RndMeth=Simplest  InputSameDT=on
  PZ : Lookup_n-D  NumberOfTableDimensions=1  BreakpointsForDimension1=breakpoints  BeginIndexSearchUsingPreviousIndexResult=on  Table=datapz  InterpMethod=Cubic spline  InternalRulePriority=Speed  RndMeth=Simplest  InputSameDT=on
  SGP4 : MATLAB Function  Commented=on  TreatAsAtomicUnit=on
  VX : Lookup_n-D  NumberOfTableDimensions=1  BreakpointsForDimension1=breakpoints  BeginIndexSearchUsingPreviousIndexResult=on  Table=datavx  InterpMethod=Cubic spline  InternalRulePriority=Speed  RndMeth=Simplest  InputSameDT=on
  VY : Lookup_n-D  NumberOfTableDimensions=1  BreakpointsForDimension1=breakpoints  BeginIndexSearchUsingPreviousIndexResult=on  Table=datavy  InterpMethod=Cubic spline  InternalRulePriority=Speed  RndMeth=Simplest  InputSameDT=on
  VZ : Lookup_n-D  NumberOfTableDimensions=1  BreakpointsForDimension1=breakpoints  BeginIndexSearchUsingPreviousIndexResult=on  Table=datavz  InterpMethod=Cubic spline  InternalRulePriority=Speed  RndMeth=Simplest  InputSameDT=on
  (PX,PY,PZ) : Outport
  (VX,VY,VZ) : Outport  Port=2
  wires:
  PX/1 -> Mux/1
  PY/1 -> Mux/2
  PZ/1 -> Mux/3
  Mux/1 -> (PX,PY,PZ)/1
  VZ/1 -> Mux1/3
  VY/1 -> Mux1/2
  VX/1 -> Mux1/1
  Mux1/1 -> (VX,VY,VZ)/1
  JD/1 -> VZ/1, VY/1, VX/1, PX/1, PY/1, PZ/1

== system ADCS_Outline/STK Attitude Recording ==
  DCM_BE : Inport
  Mode : Inport  Port=2
  Clock : Clock
  DCM to q : MATLAB Function  TreatAsAtomicUnit=on
  MATLAB Function : MATLAB Function  TreatAsAtomicUnit=on
  Mux : Mux  Inputs=2
  Pulse Generator : DiscretePulseGenerator  PulseType=Time based  Period=180  PulseWidth=5  PhaseDelay=1e-16
  Pulse Generator1 : DiscretePulseGenerator  PulseType=Time based  PulseWidth=5  PhaseDelay=1e-16
  Subsystem : Subsystem
  Switch : Switch  Threshold=1
  wires:
  DCM to q/1(q) -> Mux/2
  Clock/1 -> Mux/1
  DCM_BE/1 -> DCM to q/1(dcm_inv)
  Mux/1 -> Subsystem/1(q_EB)
  Pulse Generator1/1 -> Switch/3
  Pulse Generator/1 -> Switch/1
  Mode/1 -> MATLAB Function/1(u)
  MATLAB Function/1(y) -> Switch/2
  Switch/1 -> Subsystem/Trigger

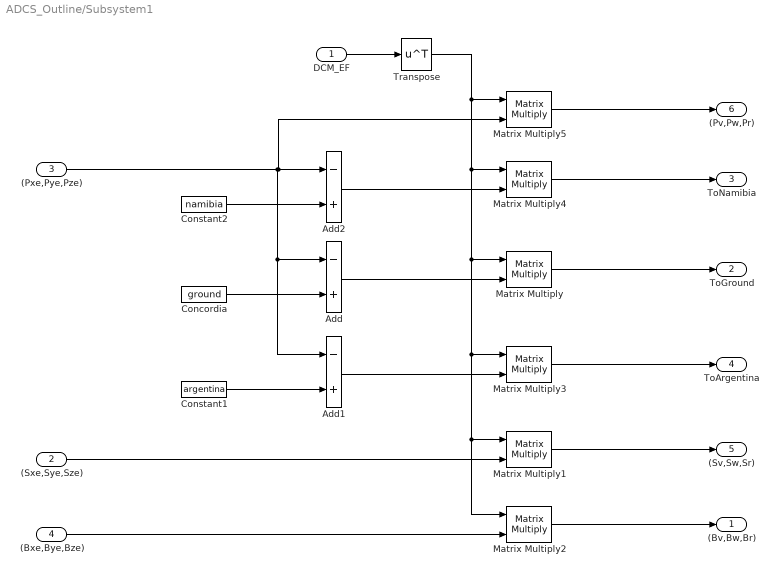
== system ADCS_Outline/Subsystem1 ==
  "DCM_EF " : Inport
  (Sxe,Sye,Sze) : Inport  Port=2
  (Pxe,Pye,Pze) : Inport  Port=3
  (Bxe,Bye,Bze) : Inport  Port=4
  Add : Sum  Inputs=-+
  Add1 : Sum  Inputs=-+
  Add2 : Sum  Inputs=-+
  Concordia : Constant  Value=ground
  Constant1 : Constant  Value=argentina
  Constant2 : Constant  Value=namibia
  Matrix Multiply{,1..5} (6 alike) : Product  Multiplication=Matrix(*)
  Transpose : Math  Operator=transpose  SaturateOnIntegerOverflow=on
  (Bv,Bw,Br) : Outport
  ToGround : Outport  Port=2
  ToNamibia : Outport  Port=3
  ToArgentina : Outport  Port=4
  (Sv,Sw,Sr) : Outport  Port=5
  (Pv,Pw,Pr) : Outport  Port=6
  wires:
  Add/1 -> Matrix Multiply/2
  "DCM_EF "/1 -> Transpose/1
  Transpose/1 -> Matrix Multiply5/1, Matrix Multiply2/1, Matrix Multiply1/1, Matrix Multiply3/1, Matrix Multiply/1, Matrix Multiply4/1
  Matrix Multiply/1 -> ToGround/1
  Concordia/1 -> Add/2
  (Sxe,Sye,Sze)/1 -> Matrix Multiply1/2
  (Bxe,Bye,Bze)/1 -> Matrix Multiply2/2
  Matrix Multiply2/1 -> (Bv,Bw,Br)/1
  Matrix Multiply1/1 -> (Sv,Sw,Sr)/1
  Matrix Multiply3/1 -> ToArgentina/1
  (Pxe,Pye,Pze)/1 -> Matrix Multiply5/2, Add2/1, Add1/1, Add/1
  Constant1/1 -> Add1/2
  Add1/1 -> Matrix Multiply3/2
  Constant2/1 -> Add2/2
  Add2/1 -> Matrix Multiply4/2
  Matrix Multiply4/1 -> ToNamibia/1
  Matrix Multiply5/1 -> (Pv,Pw,Pr)/1

== system ADCS_Outline/Sun ==
  note: MOD
  note: ECI J2000
  JD : Inport
  Constant : Constant  Value=0
  Constant1 : Constant  Value=0
  Constant2 : Constant  Value=nut80
  Fcn : Fcn  Expr=(u-2451545)/36525.0
  MATLAB Function : MATLAB Function  TreatAsAtomicUnit=on
  MATLAB Function1 : MATLAB Function  TreatAsAtomicUnit=on
  MATLAB Function2 : MATLAB Function  TreatAsAtomicUnit=on
  (SX,SY,SZ) : Outport
  wires:
  JD/1 -> Fcn/1, MATLAB Function/1(jd)
  Fcn/1 -> MATLAB Function1/2(ttt), MATLAB Function2/5(ttt)
  MATLAB Function2/1(rteme) -> (SX,SY,SZ)/1
  MATLAB Function1/1(reci) -> MATLAB Function2/3(reci)
  Constant/1 -> MATLAB Function2/1(ddpsi)
  Constant1/1 -> MATLAB Function2/2(ddeps)
  MATLAB Function/1(rsun) -> MATLAB Function1/1(rmod)
  Constant2/1 -> MATLAB Function2/4(nut80)

== system ADCS_Outline/Sun Sensors ==
  (Sx,Sy,Sz) : Inport
  Noise and Bias : Subsystem
  C(Sx,Sy,Sz) : Outport
  wires:
  (Sx,Sy,Sz)/1 -> Noise and Bias/1(In1)
  Noise and Bias/1(Out1) -> C(Sx,Sy,Sz)/1

== system ADCS_Outline/TEME to ITRF ==
  note: ateme not necessary
  note: No published values, we will assume no excess seconds to the length of day for now. https://www.iers.org/IERS/EN/Science/EarthRotation/UT1LOD.html
  note: xp and xy are retreived from https://www.iers.org/IERS/EN/DataProducts/EarthOrientationData/eop.html
  (PX,PY,PZ) : Inport
  (VX,VY,VZ) : Inport  Port=2
  JD : Inport  Port=3
  (SX,SY,SZ) : Inport  Port=4
  " " : Fcn  Expr=(u-2451545.0)/36525
  Constant : Constant  Value=[1; 1; 1]
  Constant1 : Constant  Value=2
  Constant2 : Constant  Value=0.247746*pi/3600/180
  Constant3 : Constant  Value=0.127631*pi/3600/180
  Constant4 : Constant  Value=0
  From David Vallado : MATLAB Function  TreatAsAtomicUnit=on
  Terminator : Terminator
  (Pxe,Pye,Pze) : Outport
  (Sxe,Sye,Sze) : Outport  Port=2
  (Vxe,Vye,Vze) : Outport  Port=3
  DCM_ET : Outport  Port=4
  wires:
  (PX,PY,PZ)/1 -> From David Vallado/2(rteme)
  (VX,VY,VZ)/1 -> From David Vallado/3(vteme)
  Constant/1 -> From David Vallado/4(ateme)
  From David Vallado/4(aecef) -> Terminator/1
  From David Vallado/2(recef) -> (Pxe,Pye,Pze)/1
  From David Vallado/3(vecef) -> (Vxe,Vye,Vze)/1
  Constant1/1 -> From David Vallado/10(eqeterms)
  Constant2/1 -> From David Vallado/9(yp)
  Constant3/1 -> From David Vallado/8(xp)
  Constant4/1 -> From David Vallado/7(lod)
  " "/1 -> From David Vallado/5(ttt)
  JD/1 -> From David Vallado/6(jdut1), " "/1
  (SX,SY,SZ)/1 -> From David Vallado/1(steme)
  From David Vallado/1(secef) -> (Sxe,Sye,Sze)/1
  From David Vallado/5(DCM_ET) -> DCM_ET/1

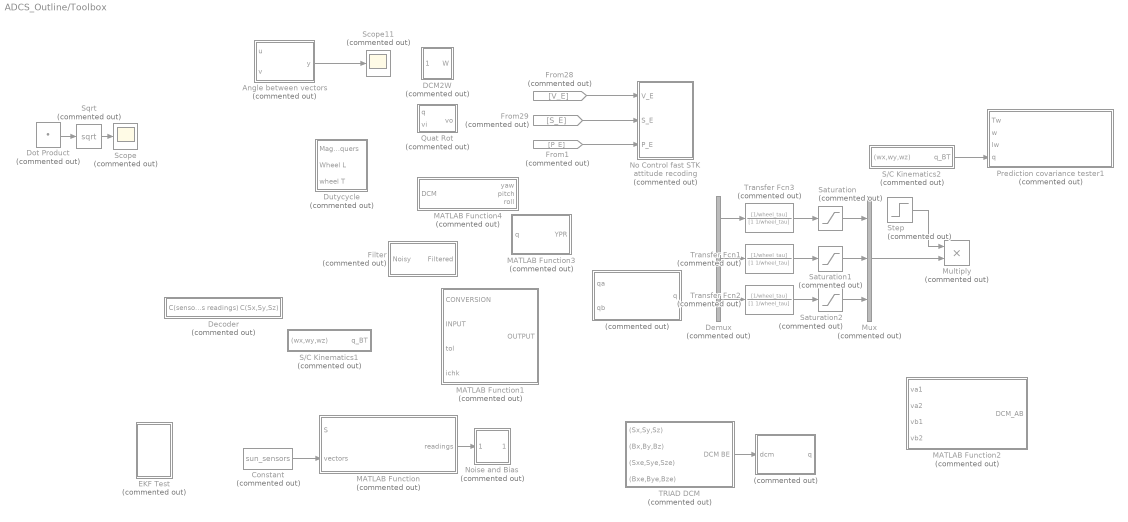
== system ADCS_Outline/Toolbox ==
  " " : MATLAB Function  Commented=on  TreatAsAtomicUnit=on
  "    " : MATLAB Function  Commented=on  TreatAsAtomicUnit=on
  Angle between vectors : MATLAB Function  Commented=on  TreatAsAtomicUnit=on
  Constant : Constant  Commented=on  Value=sun_sensors
  DCM2W : Subsystem  Commented=on
  Decoder : Subsystem  Commented=on
  Demux : Demux  Commented=on  Outputs=3
  Dot Product : DotProduct  Commented=on  InputSameDT=on  OutDataTypeStr=Inherit: Inherit via internal rule
  Dutycycle : Subsystem  Commented=on
  EKF Test : Subsystem  Commented=on
  Filter : Subsystem  Commented=on
  From1 : From  Commented=on  GotoTag=P_E
  From28 : From  Commented=on  GotoTag=V_E
  From29 : From  Commented=on  GotoTag=S_E
  MATLAB Function : MATLAB Function  Commented=on  TreatAsAtomicUnit=on
  MATLAB Function1 : MATLAB Function  Commented=on  TreatAsAtomicUnit=on
  MATLAB Function2 : MATLAB Function  Commented=on  TreatAsAtomicUnit=on
  MATLAB Function3 : MATLAB Function  Commented=on  TreatAsAtomicUnit=on
  MATLAB Function4 : MATLAB Function  Commented=on  TreatAsAtomicUnit=on
  Multiply : Product  Commented=on
  Mux : Mux  Commented=on  Inputs=3
  No Control fast STK attitude recoding : Subsystem  Commented=on
  Noise and Bias : Subsystem  Commented=on
  Prediction covariance tester1 : Subsystem  Commented=on  TreatAsAtomicUnit=on  SystemSampleTime=controller_sample_rate
  Quat Rot : Subsystem  Commented=on
  S/C Kinematics1 : Subsystem  Commented=on
  S/C Kinematics2 : Subsystem  Commented=on
  Saturation : Saturate  Commented=on  UpperLimit=wheel_saturation  LowerLimit=-wheel_saturation  ZeroCross=off
  Saturation1 : Saturate  Commented=on  UpperLimit=wheel_saturation  LowerLimit=-wheel_saturation  ZeroCross=off
  Saturation2 : Saturate  Commented=on  UpperLimit=wheel_saturation  LowerLimit=-wheel_saturation  ZeroCross=off
  Scope : Scope  Commented=on
  Scope11 : Scope  Commented=on
  Sqrt : Sqrt  Commented=on  SaturateOnIntegerOverflow=on
  Step : Step  Commented=on  Time=30  SampleTime=0
  TRIAD DCM : Subsystem  Commented=on
  Transfer Fcn1 : TransferFcn  Commented=on  Numerator=[1/wheel_tau]  Denominator=[1 1/wheel_tau]
  Transfer Fcn2 : TransferFcn  Commented=on  Numerator=[1/wheel_tau]  Denominator=[1 1/wheel_tau]
  Transfer Fcn3 : TransferFcn  Commented=on  Numerator=[1/wheel_tau]  Denominator=[1 1/wheel_tau]
  wires:
  Angle between vectors/1(y) -> Scope11/1
  From28/1 -> No Control fast STK attitude recoding/1(V_E)
  From29/1 -> No Control fast STK attitude recoding/2(S_E)
  From1/1 -> No Control fast STK attitude recoding/3(P_E)
  TRIAD DCM/1(DCM BE) -> " "/1(dcm)
  MATLAB Function/1(readings) -> Noise and Bias/1(In1)
  Constant/1 -> MATLAB Function/2(vectors)
  Demux/3 -> Transfer Fcn2/1
  Transfer Fcn1/1 -> Saturation1/1
  Step/1 -> Multiply/1
  Saturation1/1 -> Mux/2
  Transfer Fcn3/1 -> Saturation/1
  Mux/1 -> Multiply/2
  Saturation2/1 -> Mux/3
  Demux/2 -> Transfer Fcn1/1
  Saturation/1 -> Mux/1
  Demux/1 -> Transfer Fcn3/1
  Transfer Fcn2/1 -> Saturation2/1
  Dot Product/1 -> Sqrt/1
  ? -> Dot Product/1, Dot Product/2
  Sqrt/1 -> Scope/1
  S/C Kinematics2/1(q_BT) -> Prediction covariance tester1/4(q)

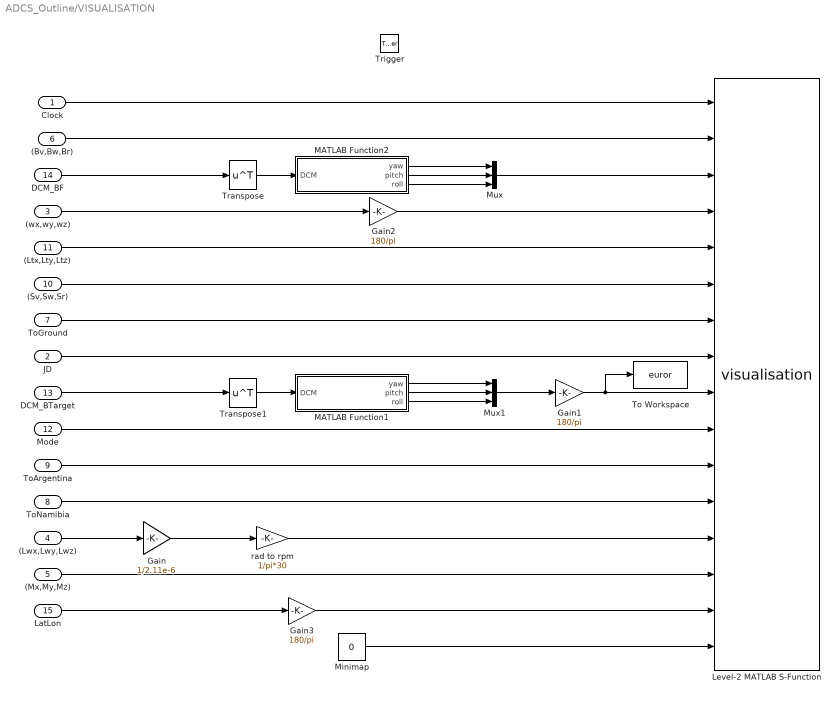
== system ADCS_Outline/VISUALISATION ==
  Clock : Inport
  JD : Inport  Port=2
  (wx,wy,wz) : Inport  Port=3
  (Lwx,Lwy,Lwz) : Inport  Port=4
  (Mx,My,Mz) : Inport  Port=5
  (Bv,Bw,Br) : Inport  Port=6
  ToGround : Inport  Port=7
  ToNamibia : Inport  Port=8
  ToArgentina : Inport  Port=9
  (Sv,Sw,Sr) : Inport  Port=10
  (Ltx,Lty,Ltz) : Inport  Port=11
  Mode : Inport  Port=12
  DCM_BTarget : Inport  Port=13
  DCM_BF : Inport  Port=14
  LatLon : Inport  Port=15
  Trigger : TriggerPort  VariantControl=Variant  PortDimensions=1
  Gain : Gain  Gain=1/2.11e-6
  Gain1 : Gain  Gain=180/pi
  Gain2 : Gain  Gain=180/pi
  Gain3 : Gain  Gain=180/pi
  Level-2 MATLAB S-Function : M-S-Function  FunctionName=visualisation  Parameters=Orbit
  MATLAB Function1 : MATLAB Function  TreatAsAtomicUnit=on
  MATLAB Function2 : MATLAB Function  TreatAsAtomicUnit=on
  Minimap : Constant  Value=0
  Mux : Mux  Inputs=3
  Mux1 : Mux  Inputs=3
  To Workspace : ToWorkspace  VariableName=euror  SampleTime=-1
  Transpose : Math  Operator=transpose  SaturateOnIntegerOverflow=on
  Transpose1 : Math  Operator=transpose  SaturateOnIntegerOverflow=on
  rad to rpm : Gain  Gain=1/pi*30
  wires:
  Mux/1 -> Level-2 MATLAB S-Function/3
  Clock/1 -> Level-2 MATLAB S-Function/1
  (Bv,Bw,Br)/1 -> Level-2 MATLAB S-Function/2
  (Sv,Sw,Sr)/1 -> Level-2 MATLAB S-Function/6
  Gain2/1 -> Level-2 MATLAB S-Function/4
  ToGround/1 -> Level-2 MATLAB S-Function/7
  JD/1 -> Level-2 MATLAB S-Function/8
  (Ltx,Lty,Ltz)/1 -> Level-2 MATLAB S-Function/5
  DCM_BF/1 -> Transpose/1
  Mux1/1 -> Gain1/1
  Gain1/1 -> To Workspace/1, Level-2 MATLAB S-Function/9
  Mode/1 -> Level-2 MATLAB S-Function/10
  ToArgentina/1 -> Level-2 MATLAB S-Function/11
  ToNamibia/1 -> Level-2 MATLAB S-Function/12
  (wx,wy,wz)/1 -> Gain2/1
  Gain/1 -> rad to rpm/1
  (Lwx,Lwy,Lwz)/1 -> Gain/1
  rad to rpm/1 -> Level-2 MATLAB S-Function/13
  (Mx,My,Mz)/1 -> Level-2 MATLAB S-Function/14
  LatLon/1 -> Gain3/1
  Gain3/1 -> Level-2 MATLAB S-Function/15
  Minimap/1 -> Level-2 MATLAB S-Function/16
  MATLAB Function1/1(yaw) -> Mux1/1
  MATLAB Function1/2(pitch) -> Mux1/2
  MATLAB Function1/3(roll) -> Mux1/3
  MATLAB Function2/1(yaw) -> Mux/1
  MATLAB Function2/2(pitch) -> Mux/2
  MATLAB Function2/3(roll) -> Mux/3
  Transpose/1 -> MATLAB Function2/1(DCM)
  DCM_BTarget/1 -> Transpose1/1
  Transpose1/1 -> MATLAB Function1/1(DCM)

== system ADCS_Outline/wheel speed feedback ==
  (Lwx,Lwy,Lwz) : Inport
  Noise and Bias : Subsystem
  Lwheel : Outport
  C_Lwheel : Outport  Port=2
  wires:
  (Lwx,Lwy,Lwz)/1 -> Lwheel/1, Noise and Bias/1(In1)
  Noise and Bias/1(Out1) -> C_Lwheel/1
